simulink model "antiwindup_main"  (R2015a)
settings: Solver=ode45  StartTime=0.0  StopTime=10.0  RelTol=1e-3
settings Model: Creator=teme  LastModifiedBy=teme

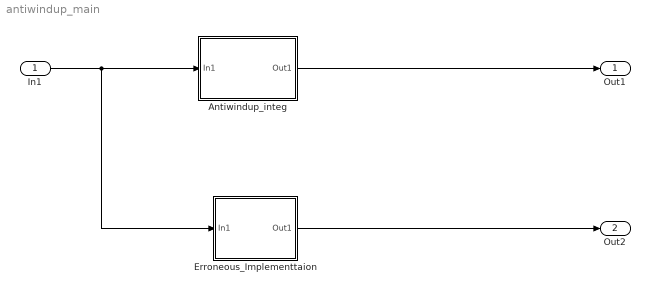
== system antiwindup_main ==
  In1 : Inport
  Antiwindup_integ : Subsystem
  Erroneous_Implementtaion : Subsystem
  Out1 : Outport
  Out2 : Outport  Port=2
  wires:
  In1/1 -> Erroneous_Implementtaion/1(In1), Antiwindup_integ/1(In1)
  Antiwindup_integ/1(Out1) -> Out1/1
  Erroneous_Implementtaion/1(Out1) -> Out2/1

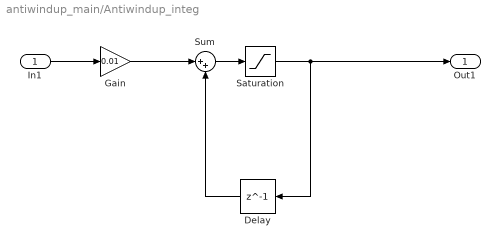
== system antiwindup_main/Antiwindup_integ ==
  In1 : Inport
  Delay : Delay  DelayLength=1  InitialCondition=0
  Gain : Gain  Gain=0.01
  Saturation : Saturate
  Sum : Sum  Inputs=|++
  Out1 : Outport
  wires:
  Sum/1 -> Saturation/1
  Gain/1 -> Sum/1
  Saturation/1 -> Out1/1, Delay/1
  Delay/1 -> Sum/2
  In1/1 -> Gain/1

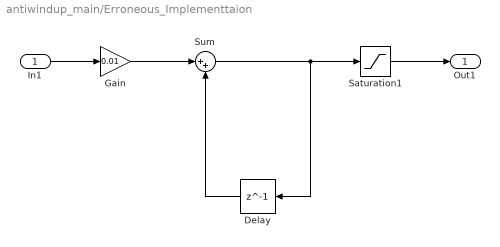
== system antiwindup_main/Erroneous_Implementtaion ==
  In1 : Inport
  Delay : Delay  DelayLength=1  InitialCondition=0
  Gain : Gain  Gain=0.01
  Saturation1 : Saturate
  Sum : Sum  Inputs=|++
  Out1 : Outport
  wires:
  In1/1 -> Gain/1
  Delay/1 -> Sum/2
  Gain/1 -> Sum/1
  Sum/1 -> Saturation1/1, Delay/1
  Saturation1/1 -> Out1/1
